simulink model "APSv3"  (R2020b)
settings: Solver=FixedStepDiscrete  StartTime=0.0  StopTime=Tmax  FixedStep=Ts  RelTol=1e-3
PreLoadFcn:
  | ROSconfig
  | wptsSignalSetup
PostLoadFcn:
  | configParameters
InitFcn:
  | configParameters
StartFcn:
  | gazeboSetup
StopFcn:
  | gazeboReset
  | goalreset
  | loadResults
model workspace (MAT data in the model file):
  idx = 1
  y = Simulink.Parameter
  y.DataType = 'auto'
  y.Dimensions = [0 0]
values from neighbouring files (symbols this model uses):
  distError = sqrt((initX^2)+(initY^2))    [config_APS_Turb.m]
  dynamicPlume = 0    [config_APS_Turb.m]
  init = [initX - 5,initY]    [config_APS_Turb.m]
  MaxC = max(max(max(PlumeD)))    [config_APS_Turb.m]
  N = 8    [config_APS_Turb.m]
  n = [n; i*(2*pi/N)]    [config_APS_Turb.m]
  Res = 1    [config_APS_Turb.m]
  Shrink = 1/Expand    [config_APS_Turb.m]
undefined symbols (not defined in the file or in its folder): angmax, Angular, concDetectionAccuracy, DiscIntNeverNeededParam, distThresh, Expand, get, hot, Kd, Ki, Kp, LimitSize, Linear, OffsetY, PlumeD, ResX, ResY, sensorDist, sourceAccuracy, T, Tmax, Ts, vmax, wgain
libraries: simulink x18, dspindex x8, dspswit3 x6, robotlib x3, dspsnks4 x3, sm_lib x2, nesl_utility x1, dspsigops x1, mobileRoboticsLib x1
(part 1 of 2)
PauseFcn:
  | gazeboPause
settings Model: OrderedModelArguments=off  Creator=ty  LastModifiedBy=Tyreeses'
settings SolverCC: AlgebraicLoopSolver=LineSearch
settings DataIOCC: ExternalInput=[r, b]  SaveFormat=Array  SaveState=on  InspectSignalLogs=on  ReturnWorkspaceOutputs=off  StateSaveName=wpts
settings DebuggingCC: ArithmeticOperatorsInVariantConditions=warning
settings SFSimCC: SimUseLocalCustomCode=off  CustomCodeUndefinedFunction=UseInterfaceOnly
settings RTWCC: RTWUseLocalCustomCode=off
settings SimMechanicsCC: VisOnUpdateDiagram=on  VisDuringSimulation=on  DefaultBodyColor=[.877 0 0]
settings ExplorerConfigSet: SimMechanicsOpenEditorOnUpdate=off  InternalSimMechanicsExplorerSettings="<ExplorerConfiguration><canonicalview>default</canonicalview><AnimationSetting><BasePlaybackSpeed>1.0</BasePlaybackSpeed><PlaybackSpeedFactor>4.0</PlaybackSpeedFactor></AnimationSetting><TilePanel><TileInfo><Tiles Columns=\"2\" Count=\"4\" Rows=\"2\"><Column Weight=\"0.5\"/><Column Weight=\"0.5\"/><Row Weight=\"0.5\"/><Row Weight=\"0.5\"/><Tile Height=\"1\" Width=\"1\" X=\"0\" Y=\"0\"/><Tile Height=\"1\" Width=\"1\" X=\"0\" Y=\"1\"/><Tile Height=\"1\" Width=\"1\" X=\"1\" Y=\"0\"/><Tile Height=\"1\" Width=\"1\" X=\"1\" Y=\"1\"/></Tiles></TileInfo><SceneInfo><SceneViewer><BGColor><R>0.60000002384185791</R><G>0.60000002384185791</G><B>0.60000002384185791</B></BGColor><Camera><DoPerspective>off</DoPerspective><Position><X>0.523539858098702515</X><Y>-0.526832295844210763</Y><Z>1.31558763938248235</Z></Position><Center><X>0.523539858098702515</X><Y>-0.526832295844210763</Y><Z>0.315587639382482354</Z></Center><Up><X>0</X><Y>1</Y><Z>-0</Z></Up><ViewLimDist>1</ViewLimDist><YLim>8.09056691591361421</YLim><XLim>11.4549610789668002</XLim></Camera></SceneViewer><SceneViewer><BGColor><R>0.60000002384185791</R><G>0.60000002384185791</G><B>0.60000002384185791</B></BGColor><Camera><DoPerspective>off</DoPerspective><Position><X>-1.00000000034924597</X><Y>-0.123102183445061519</Y><Z>0.275798201199813964</Z></Position><Center><X>-3.49245965480804443e-10</X><Y>-0.123102183445061519</Y><Z>0.275798201199813964</Z></Center><Up><X>0</X><Y>0</Y><Z>1</Z></Up><ViewLimDist>1</ViewLimDist><YLim>3.47753295219900371</YLim><XLim>4.92363576400452985</XLim></Camera></SceneViewer><SceneViewer><BGColor><R>0.60000002384185791</R><G>0.60000002384185791</G><B>0.60000002384185791</B></BGColor><Camera><DoPerspective>off</DoPerspective><Position><X>0.692144908773628886</X><Y>-0.692774488443842151</Y><Z>0.641997243049143074</Z></Position><Center><X>0.114794639584003433</X><Y>-0.115424219254216046</Y><Z>0.0646469738595174259</Z></Center><Up><X>-0.408248290463863073</X><Y>0.408248290463863073</Y><Z>0.816496580927726145</Z></Up><ViewLimDist>1</ViewLimDist><YLim>6.0070720394774666</YLim><XLim>8.50506239252750262</XLim></Camera></SceneViewer><SceneViewer><BGColor><R>0.60000002384185791</R><G>0.60000002384185791</G><B>0.60000002384185791</B></BGColor><Camera><DoPerspective>off</DoPerspective><Position><X>0.0489598554332313918</X><Y>-0.287272213681231237</Y><Z>1.31558770067272501</Z></Position><Center><X>0.0489598554332313918</X><Y>-0.287272213681231237</Y><Z>0.315587700672725013</Z></Center><Up><X>0</X><Y>1</Y><Z>-0</Z></Up><ViewLimDist>1</ViewLimDist><YLim>2.42704539801906094</YLim><XLim>3.4363118011556999</XLim></Camera></SceneViewer></SceneInfo></TilePanel><MechEditorPanel><Cameras><Camera><Id>Camera1</Id><Value><Name>TopCamera1</Name><NativeCamera><PositionKeyframeSet><Keyframe><Time>+0.0000000000000000e+00</Time><Value><X>+2.1442706964244174e-01</X><Y>+2.3082412087368320e-01</Y><Z>+8.5801428178680403e+00</Z></Value></Keyframe></PositionKeyframeSet><CenterKeyframeSet><Keyframe><Time>+0.0000000000000000e+00</Time><Value><X>+1.7666087274208450e-01</X><Y>+1.6219238056249624e-01</Y><Z>+3.9566976367888529e-01</Z></Value></Keyframe></CenterKeyframeSet><UpVectorKeyframeSet><Keyframe><Time>+0.0000000000000000e+00</Time><Value><X>-1.4536948631457236e-02</X><Y>+9.9985973958876295e-01</Y><Z>-8.3173477730344968e-03</Z></Value></Keyframe></UpVectorKeyframeSet></NativeCamera></Value></Camera></Cameras><GfxPanelCameraMap/><VideoCreator><PlaybackSpeedRatio>1.0</PlaybackSpeedRatio><FrameRate>30</FrameRate><VideoFormat>Motion JPEG AVI</VideoFormat><FrameSize>auto</FrameSize></VideoCreator></MechEditorPanel></ExplorerConfiguration>"

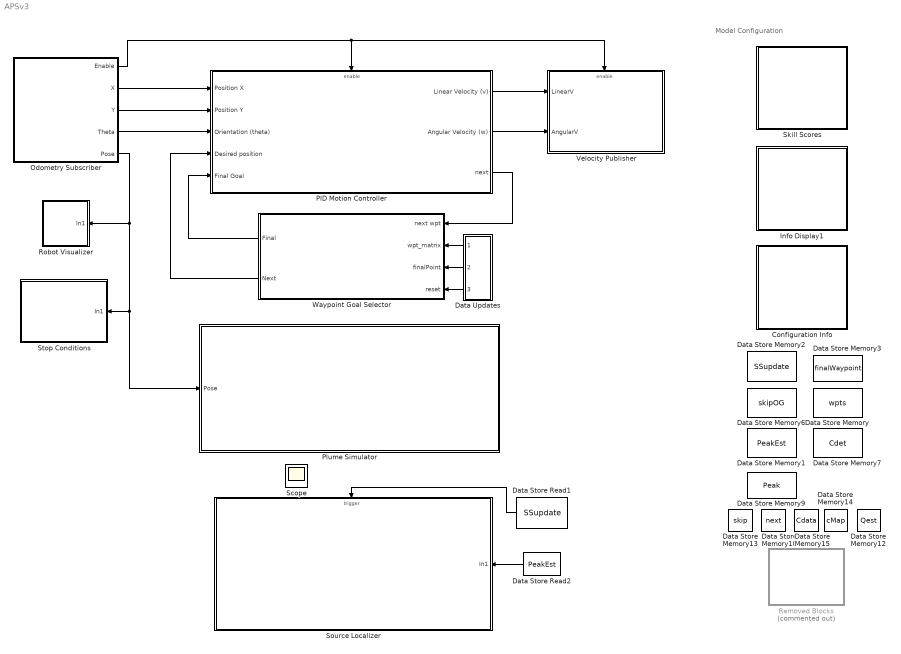
== system APSv3 ==
  note: Model Configuration
  Configuration Info : Subsystem
  Data Store Memory : DataStoreMemory  DataStoreName=wpts  ReadBeforeWriteMsg=warning  WriteAfterWriteMsg=warning  WriteAfterReadMsg=warning  InitialValue=waypoints  VectorParams1D=off  ShowAdditionalParam=off
  Data Store Memory1 : DataStoreMemory  DataStoreName=PeakEst  ReadBeforeWriteMsg=warning  WriteAfterWriteMsg=warning  WriteAfterReadMsg=warning  InitialValue=[25 25]  VectorParams1D=off  ShowAdditionalParam=off
  Data Store Memory10 : DataStoreMemory  DataStoreName=next  ReadBeforeWriteMsg=warning  WriteAfterWriteMsg=warning  WriteAfterReadMsg=warning  ShowAdditionalParam=off
  Data Store Memory12 : DataStoreMemory  DataStoreName=Qest  ReadBeforeWriteMsg=warning  WriteAfterWriteMsg=warning  WriteAfterReadMsg=warning  ShowAdditionalParam=off
  Data Store Memory13 : DataStoreMemory  DataStoreName=skip  ReadBeforeWriteMsg=warning  WriteAfterWriteMsg=warning  WriteAfterReadMsg=warning  ShowAdditionalParam=off
  Data Store Memory14 : DataStoreMemory  DataStoreName=cMap  ReadBeforeWriteMsg=warning  WriteAfterWriteMsg=warning  WriteAfterReadMsg=warning  InitialValue=zeros(size(PlumeD,1),size(PlumeD,2))  VectorParams1D=off  ShowAdditionalParam=off
  Data Store Memory15 : DataStoreMemory  DataStoreName=Cdata  ReadBeforeWriteMsg=warning  WriteAfterWriteMsg=warning  WriteAfterReadMsg=warning  InitialValue=ones(N+1,1)  ShowAdditionalParam=off  OutDataTypeStr=double
  Data Store Memory2 : DataStoreMemory  DataStoreName=SSupdate  ReadBeforeWriteMsg=warning  WriteAfterWriteMsg=warning  WriteAfterReadMsg=warning  InitialValue=1  ShowAdditionalParam=off  OutDataTypeStr=boolean
  Data Store Memory3 : DataStoreMemory  DataStoreName=finalWaypoint  ReadBeforeWriteMsg=warning  WriteAfterWriteMsg=warning  WriteAfterReadMsg=warning  InitialValue=finalPoint  ShowAdditionalParam=off  OutDataTypeStr=double
  Data Store Memory6 : DataStoreMemory  DataStoreName=skipOG  ReadBeforeWriteMsg=warning  WriteAfterWriteMsg=warning  WriteAfterReadMsg=warning  ShowAdditionalParam=off
  Data Store Memory7 : DataStoreMemory  DataStoreName=Cdet  ReadBeforeWriteMsg=warning  WriteAfterWriteMsg=warning  WriteAfterReadMsg=warning  ShowAdditionalParam=off
  Data Store Memory9 : DataStoreMemory  DataStoreName=Peak  ReadBeforeWriteMsg=warning  WriteAfterWriteMsg=warning  WriteAfterReadMsg=warning  InitialValue=[0,0]  ShowAdditionalParam=off
  Data Store Read1 : DataStoreRead  DataStoreName=SSupdate
  Data Store Read2 : DataStoreRead  DataStoreName=PeakEst
  Data Updates : Subsystem
  Info Display1 : Subsystem
  Odometry Subscriber : Subsystem
  PID Motion Controller : Subsystem
  Plume Simulator : Subsystem
  Removed Blocks : Subsystem  Commented=on
  Robot Visualizer : Subsystem
  Skill Scores : Subsystem
  Source Localizer : Subsystem  TreatAsAtomicUnit=on
  Stop Conditions : Subsystem
  Velocity Publisher : Subsystem
  Waypoint Goal Selector : Subsystem
  Scope : Scope
  wires:
  PID Motion Controller/1(Linear Velocity (v)) -> Velocity Publisher/1(LinearV)
  PID Motion Controller/2(Angular Velocity (w)) -> Velocity Publisher/2(AngularV)
  PID Motion Controller/3(next) -> Waypoint Goal Selector/1(next wpt)
  Waypoint Goal Selector/1(Final) -> PID Motion Controller/5(Final Goal)
  Waypoint Goal Selector/2(Next) -> PID Motion Controller/4(Desired position)
  Data Store Read2/1 -> Source Localizer/1(In1)
  Data Store Read1/1 -> Source Localizer/Trigger
  Data Updates/1(Out1) -> Waypoint Goal Selector/2(wpt_matrix)
  Data Updates/2(Out2) -> Waypoint Goal Selector/3(finalPoint)
  Data Updates/3(Out3) -> Waypoint Goal Selector/4(reset)
  Odometry Subscriber/1(Enable) -> Velocity Publisher/Enable, PID Motion Controller/Enable
  Odometry Subscriber/5(Pose) -> Plume Simulator/1(Pose), Stop Conditions/1(In1), Robot Visualizer/1(In1)
  Odometry Subscriber/2(X) -> PID Motion Controller/1(Position X)
  Odometry Subscriber/3(Y) -> PID Motion Controller/2(Position Y)
  Odometry Subscriber/4(Theta) -> PID Motion Controller/3(Orientation (theta))

== system APSv3/Configuration Info ==
  note: Nodes :
      | Publishers:
      | /sim_p3at/cmd_vel
      | /toggle_led
      | Subscribers:
      | /sim_p3at/odom
      | Messages:
      | geometry_msgs/Twist
      | std_msgs/Empty
  note: Startup Programs :
      | roscore
      | roslaunch nre_p3at p3at.gazebo.launch (starts Gazebo and /sim_p3at Nodes)
      | Arduino: ledtest3.ino
      | rosrun rosserial_python serial_node.py /dev/ttyACM0
      | MATLAB: (Simulink project)
  note: SS Parameters :
      | Expansion Constant: 2
  note: Plume Parameters :
      |
      | Diffusion constant (m2/s): c_diff = .8
      |
      | Advection velocity values (m/s): ux = 0 uy = 0 uz = 0.2
      |
      | Simulation Time (seconds): T = 10
      |
      | Domain dimensions (meters): L = 50 B = 50 H = 5
  "Counter " : Subsystem  Commented=on
  Floating Scope : Scope  Commented=on
      settings: Floating=on
  MechanismConfiguration : sm_lib/Utilities/Mechanism Configuration  UniformGravity=Constant  GravityVector=[0 0 -9.80665]  GravityUnits=m/s^2  LinearizationDelta=0.01
  Solver Configuration : nesl_utility/Solver Configuration  PhysicalDomain=network_engine_domain  SubClassName=solver  LeftPortType=input  RightPortType=generic  Accelerate=off  Tones=[]  Harmonics=[]  SimulateNoise=off  Profile=off  UseLocalSampling=off  EnableSwitchedLinearOptims=on  FrequencyDomain=off  UseCCode=off  RelTol=0.001  AbsTol=1e-06  MinStep=1e-09  ToWorkspace=off  RevertToSquareIcSolve=off  NumHomotopyIterations=100  PhasorMode=off  PhasorModeNumHarmonics=1  DoDC=on  ResidualTolerance=1e-09  UseLocalSolver=on  LocalSolverChoice=NE_BACKWARD_EULER_ADVANCER  LocalSolverSampleTime=Ts  DoFixedCost=on  MaxNonlinIter=3  MaxModeIter=2  LinearAlgebra=Sparse  DelaysMemoryBudget=1024  AutomaticFiltering=on  FilteringTimeConstant=0.01
  World : sm_lib/Frames and Transforms/World Frame
  connections:
  MechanismConfiguration/RConn1 -- World/RConn1 -- Solver Configuration/RConn1

== system APSv3/Data Updates ==
  Data Store Read : DataStoreRead  DataStoreName=wpts
  Data Store Read3 : DataStoreRead  DataStoreName=finalWaypoint
  Data Store Read5 : DataStoreRead  DataStoreName=SSupdate
  Data Store Write1 : DataStoreWrite  DataStoreName=finalWaypoint
  Demux : Demux  Outputs=2
  Probe : Probe  ProbeWidth=off  ProbeSampleTime=off  ProbeComplexSignal=off  ProbeSignalDimensions=on
  Terminator : Terminator
  Out1 : Outport  VectorParamsAs1DForOutWhenUnconnected=off
  Out2 : Outport  Port=2  VectorParamsAs1DForOutWhenUnconnected=off
  Out3 : Outport  Port=3  VectorParamsAs1DForOutWhenUnconnected=off
  wires:
  Data Store Read3/1 -> Out2/1
  Data Store Read/1 -> Out1/1, Probe/1
  Probe/1 -> Demux/1
  Demux/1 -> Data Store Write1/1
  Demux/2 -> Terminator/1
  Data Store Read5/1 -> Out3/1

== system APSv3/Info Display1 ==
  Clock : Clock
      settings: Decimation=2
  Constant : Constant  Value=[0 OffsetY]
  Constant1 : Constant  Value=MaxC
  Data Store Read : DataStoreRead  DataStoreName=PeakEst
  Data Store Read1 : DataStoreRead  DataStoreName=Peak
  Data Store Read3 : DataStoreRead  DataStoreName=Cdet
  Data Store Read4 : DataStoreRead  DataStoreName=Qest
  Detected Concentration Levels : DashboardScope  ShowInitialText=off  Ymin=0  Ymax=1000
  Display{,1..5} (6 alike) : Display
  Localization Error : DashboardScope  Ymin=0  Ymax=1.25  LegendPosition=Hide
  Sum1 : Sum
  To Workspace : ToWorkspace  VariableName=Tm  SampleTime=-1
      settings: MaxDataPoints=100
  wires:
  Data Store Read1/1 -> Display/1
  Data Store Read/1 -> Sum1/1
  Data Store Read4/1 -> Display3/1
  Constant1/1 -> Display2/1
  Clock/1 -> To Workspace/1, Display1/1
  Data Store Read3/1 -> Display5/1
  Constant/1 -> Sum1/2
  Sum1/1 -> Display4/1

== system APSv3/Odometry Subscriber ==
  Odometry Conversion : Subsystem
  Subscribe1 : robotlib/Subscribe  SourceLibraryInfo=This block requires Robotics System Toolbox  topicSource=Select from ROS network  topic=/sim_p3at/odom  messageType=nav_msgs/Odometry  sampleTime=-1  messageQueueLength=51
  Enable : Outport  VectorParamsAs1DForOutWhenUnconnected=off
  X : Outport  Port=2  VectorParamsAs1DForOutWhenUnconnected=off
  Y : Outport  Port=3  VectorParamsAs1DForOutWhenUnconnected=off
  Theta : Outport  Port=4  VectorParamsAs1DForOutWhenUnconnected=off
  Pose : Outport  Port=5  VectorParamsAs1DForOutWhenUnconnected=off
  wires:
  Subscribe1/1 -> Enable/1
  Subscribe1/2 -> Odometry Conversion/1(In1)
  Odometry Conversion/3(Out3) -> Theta/1
  Odometry Conversion/4(pose) -> Pose/1
  Odometry Conversion/1(<X>) -> X/1
  Odometry Conversion/2(<Y>) -> Y/1

== system APSv3/PID Motion Controller ==
  Position X : Inport
  Position Y : Inport  Port=2
  Orientation (theta) : Inport  Port=3
  Desired position : Inport  Port=4
  Final Goal : Inport  Port=5
  Enable : EnablePort
  Compare To Zero1 : simulink/Logic and Bit Operations/Compare To Zero  relop=>  OutDataTypeStr=boolean
  Constant3 : Constant  Value=0
  Data Store Write : DataStoreWrite  DataStoreName=SSupdate
  Data Store Write1 : DataStoreWrite  DataStoreName=next
  Initialize Goal : Subsystem
  PID Calculations : Subsystem
  Switch1 : Switch  Criteria=u2 ~= 0
  Linear Velocity (v) : Outport  VectorParamsAs1DForOutWhenUnconnected=off
  Angular Velocity (w) : Outport  Port=2  VectorParamsAs1DForOutWhenUnconnected=off
  next : Outport  Port=3  VectorParamsAs1DForOutWhenUnconnected=off
  wires:
  Switch1/1 -> Angular Velocity (w)/1
  Compare To Zero1/1 -> Data Store Write1/1, next/1
  Constant3/1 -> Switch1/1
  Final Goal/1 -> Data Store Write/1
  PID Calculations/2(Out2) -> Compare To Zero1/1, Switch1/2
  Desired position/1 -> Initialize Goal/1(In1)  "SP"
  Position Y/1 -> PID Calculations/2(In2)
  Position X/1 -> PID Calculations/3(In3)
  Orientation (theta)/1 -> PID Calculations/4(In4)
  PID Calculations/1(Out1) -> Linear Velocity (v)/1
  PID Calculations/3(Out3) -> Switch1/3
  Initialize Goal/1(Out1) -> PID Calculations/1(SP)

== system APSv3/Plume Simulator ==
  Pose : Inport
  C(t,x,y) : Subsystem
  Peak Selector : Subsystem
  Plume Model Data Simulator : Subsystem
  Terminator : Terminator
  Terminator1 : Terminator
  wires:
  C(t,x,y)/1(z(t)) -> Peak Selector/1(In1)
  Peak Selector/2(Peak C) -> Terminator1/1
  Peak Selector/1(Peak Pose) -> Terminator/1
  Pose/1 -> Plume Model Data Simulator/1(In2)
  Plume Model Data Simulator/2(t) -> C(t,x,y)/2(time)
  Plume Model Data Simulator/1(C) -> C(t,x,y)/1(c)
  Plume Model Data Simulator/3(MaxPose) -> C(t,x,y)/3(In1)

== system APSv3/Removed Blocks ==
  Constant3 : Constant  Value=MaxC
  Data Store Memory11 : DataStoreMemory  DataStoreName=locError  ReadBeforeWriteMsg=warning  WriteAfterWriteMsg=warning  WriteAfterReadMsg=warning  ShowAdditionalParam=off
  Data Store Memory16 : DataStoreMemory  DataStoreName=finalPoint  ReadBeforeWriteMsg=warning  WriteAfterWriteMsg=warning  WriteAfterReadMsg=warning  ShowAdditionalParam=off
  Data Store Memory4 : DataStoreMemory  DataStoreName=OG  ReadBeforeWriteMsg=warning  WriteAfterWriteMsg=warning  WriteAfterReadMsg=warning  InitialValue=[0 0]  ShowAdditionalParam=off
  Data Store Memory5 : DataStoreMemory  DataStoreName=DT  ReadBeforeWriteMsg=warning  WriteAfterWriteMsg=warning  WriteAfterReadMsg=warning  InitialValue=[0]  VectorParams1D=off  ShowAdditionalParam=off
  Data Store Memory8 : DataStoreMemory  DataStoreName=Cmax  ReadBeforeWriteMsg=warning  WriteAfterWriteMsg=warning  WriteAfterReadMsg=warning  InitialValue=MaxC  ShowAdditionalParam=off
  Display2 : Display  Commented=on
  Dynamic Plume Concentrations : Subsystem  Commented=on
  Gain : Gain  Commented=on  Gain=1/Ts
  Rounding Function2 : Rounding  Commented=on  Operator=ceil
  Saturation : Saturate  Commented=on  UpperLimit=T/Ts  LowerLimit=1
  Subsystem : Subsystem  Commented=on
  Terminator : Terminator  Commented=on
  To Workspace3 : ToWorkspace  VariableName=Cmax1  SaveFormat=Timeseries  SampleTime=-1
  wires:
  Gain/1 -> Rounding Function2/1
  Dynamic Plume Concentrations/1(peak) -> Subsystem/1(In1)
  Saturation/1 -> Dynamic Plume Concentrations/1(DT)
  Dynamic Plume Concentrations/2(plume) -> Terminator/1
  Subsystem/1(Out1) -> Display2/1
  Rounding Function2/1 -> Saturation/1  "u"
  Constant3/1 -> To Workspace3/1

== system APSv3/Robot Visualizer ==
  In1 : Inport
  Constant1 : Constant
  Current Origin : dspindex/Variable Selector  NumInputs=1  rowsOrCols=Rows  IdxMode=Variable  Elements=[1 3]  ZerOneIdxMode=One-based  errmode=Clip Index  FillMode=off  FillValues=0
  Data Store Read : DataStoreRead  DataStoreName=next
  Data Store Read4 : DataStoreRead  DataStoreName=wpts
  Robot Visualizer : mobileRoboticsLib/Environments/Robot Visualizer  Priority=99  robotRadius=.34  mapName=gasMap  showTrajectory=on  hasWaypoints=on  hasLidar=off  sensorOffset=[ 0 0 ]  scanAngles=0  hasObjDetector=off  objDetectorOffset=[ 0,0 ]  objDetectorAngle=0  objDetectorFOV=0  objDetectorMaxRange=0  objectColors=[1,0,0;0,1,0;0,0,1]  objectMarkers='s'
  To Workspace : ToWorkspace  VariableName=goalpoints  SampleTime=-1
      settings: Save2DSignal=2-D array (concatenate along first dimension)
  Triggered To Workspace : dspsnks4/Triggered To Workspace  TriggerType=Rising edge  VariableName=pathUpdates  Buffer=1000  Save2DMode=3-D array (concatenate along third dimension)
      settings: SourceProductBaseCode=DS  FixptAsFi=off
  wires:
  In1/1 -> Robot Visualizer/1
  Data Store Read4/1 -> To Workspace/1, Current Origin/1, Robot Visualizer/2
  Data Store Read/1 -> Triggered To Workspace/Trigger
  Constant1/1 -> Current Origin/2
  Current Origin/1 -> Triggered To Workspace/1

== system APSv3/Skill Scores ==
  Location Estimate (SL) : Subsystem
  Source Estimate (SQ) : Subsystem

== system APSv3/Source Localizer ==
  In1 : Inport
  Trigger : TriggerPort  VariantControl=Variant  InitialTriggerSignalState=positive  PortDimensions=1
  Data Store Read : DataStoreRead  DataStoreName=wpts
  Data Store Write : DataStoreWrite  DataStoreName=wpts
  Path Search Update : Subsystem
  wires:
  Data Store Read/1 -> Path Search Update/1(In1)
  In1/1 -> Path Search Update/2(In2)
  Path Search Update/1(Out1) -> Data Store Write/1

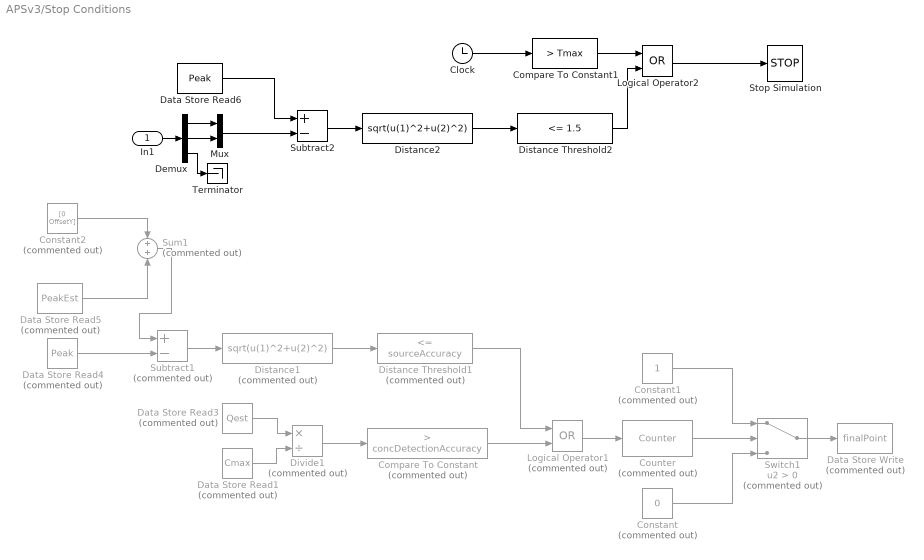
== system APSv3/Stop Conditions ==
  In1 : Inport
  Clock : Clock
  Compare To Constant : simulink/Logic and Bit Operations/Compare To Constant  Commented=on  relop=>  const=concDetectionAccuracy  OutDataTypeStr=boolean
  Compare To Constant1 : simulink/Logic and Bit Operations/Compare To Constant  relop=>  const=Tmax  OutDataTypeStr=boolean
  Constant : Constant  Commented=on  Value=0
  Constant1 : Constant  Commented=on
  Constant2 : Constant  Commented=on  Value=[0 OffsetY]
  Counter : dspswit3/Counter  Commented=on  Direction=Up  CountEvent=Rising edge  CounterSize=User defined  MaxCount=255  InitialCount=0  Output=Count  HitValue=32  ResetInput=off  SamplesPerFrame=1  Ts=1  CntDtype=double  HitDtype=Logical
  Data Store Read1 : DataStoreRead  Commented=on  DataStoreName=Cmax
  Data Store Read3 : DataStoreRead  Commented=on  DataStoreName=Qest
  Data Store Read4 : DataStoreRead  Commented=on  DataStoreName=Peak
  Data Store Read5 : DataStoreRead  Commented=on  DataStoreName=PeakEst
  Data Store Read6 : DataStoreRead  DataStoreName=Peak
  Data Store Write : DataStoreWrite  Commented=on  DataStoreName=finalPoint
  Demux : Demux  Outputs=3
  Distance Threshold1 : simulink/Logic and Bit Operations/Compare To Constant  Commented=on  relop=<=  const=sourceAccuracy  OutDataTypeStr=boolean
  Distance Threshold2 : simulink/Logic and Bit Operations/Compare To Constant  relop=<=  const=1.5  OutDataTypeStr=boolean
  Distance1 : Fcn  Commented=on  Expr=sqrt(u(1)^2+u(2)^2)
  Distance2 : Fcn  Expr=sqrt(u(1)^2+u(2)^2)
  Divide1 : Product  Commented=on  Inputs=*/
  Logical Operator1 : Logic  Commented=on  Operator=OR  AllPortsSameDT=off  OutDataTypeStr=boolean
  Logical Operator2 : Logic  Operator=OR  AllPortsSameDT=off  OutDataTypeStr=boolean
  Mux : Mux  Inputs=2
  Stop Simulation : Stop
  Subtract1 : Sum  Commented=on  Inputs=+-
  Subtract2 : Sum  Inputs=+-
  Sum1 : Sum  Commented=on
  Switch1 : Switch  Commented=on  Criteria=u2 > Threshold
  Terminator : Terminator
  wires:
  Logical Operator1/1 -> Counter/1
  Compare To Constant/1 -> Logical Operator1/2
  Data Store Read3/1 -> Divide1/1
  Data Store Read5/1 -> Sum1/2
  Subtract1/1 -> Distance1/1
  Distance Threshold1/1 -> Logical Operator1/1
  Data Store Read4/1 -> Subtract1/2
  Data Store Read1/1 -> Divide1/2
  Distance1/1 -> Distance Threshold1/1
  Divide1/1 -> Compare To Constant/1
  Data Store Read6/1 -> Subtract2/1
  Subtract2/1 -> Distance2/1
  Distance2/1 -> Distance Threshold2/1
  Distance Threshold2/1 -> Logical Operator2/2
  Constant1/1 -> Switch1/1
  Constant/1 -> Switch1/3
  Counter/1 -> Switch1/2
  Switch1/1 -> Data Store Write/1
  In1/1 -> Demux/1
  Demux/1 -> Mux/1
  Demux/2 -> Mux/2
  Mux/1 -> Subtract2/2
  Demux/3 -> Terminator/1
  Constant2/1 -> Sum1/1
  Sum1/1 -> Subtract1/1
  Compare To Constant1/1 -> Logical Operator2/1
  Clock/1 -> Compare To Constant1/1
  Logical Operator2/1 -> Stop Simulation/1

== system APSv3/Velocity Publisher ==
  LinearV : Inport
  AngularV : Inport  Port=2
  Enable : EnablePort
  Blank Message : robotlib/Blank Message  SourceLibraryInfo=This block requires Robotics System Toolbox  messageType=geometry_msgs/Twist  SampleTime=-1
  Bus Assignment : BusAssignment  DialogController=Simulink.DDGSource_BusAssignment  AssignedSignals=Linear.X,Angular.Z
  Publish1 : robotlib/Publish  SourceLibraryInfo=This block requires Robotics System Toolbox  topicSource=Select from ROS network  topic=/sim_p3at/cmd_vel  messageType=geometry_msgs/Twist  messageQueueLength=105
  wires:
  AngularV/1 -> Bus Assignment/3
  Bus Assignment/1 -> Publish1/1
  LinearV/1 -> Bus Assignment/2
  Blank Message/1 -> Bus Assignment/1

== system APSv3/Waypoint Goal Selector ==
  next wpt : Inport
  wpt_matrix : Inport  Port=2
  finalPoint : Inport  Port=3
  reset : Inport  Port=4
  "Counter " : Subsystem
  Current Goal Selector : dspindex/Variable Selector  NumInputs=1  rowsOrCols=Rows  IdxMode=Variable  Elements=[1 3]  ZerOneIdxMode=One-based  errmode=Clip Index  FillMode=off  FillValues=0
  Data Store Read : DataStoreRead  DataStoreName=skipOG
  Relational Operator : RelationalOperator  Operator===  OutDataTypeStr=boolean  RndMeth=Simplest
  Skip Conditions : Subsystem
  Sum : Sum  Inputs=|++
  Final : Outport  VectorParamsAs1DForOutWhenUnconnected=off
  Next : Outport  Port=2  VectorParamsAs1DForOutWhenUnconnected=off
  wires:
  wpt_matrix/1 -> Current Goal Selector/1
  Current Goal Selector/1 -> Next/1
  "Counter "/1(Out1) -> Sum/1
  next wpt/1 -> Skip Conditions/1(In1), "Counter "/1(In1)
  Relational Operator/1 -> Final/1
  finalPoint/1 -> Relational Operator/1
  reset/1 -> "Counter "/2(In2)
  Data Store Read/1 -> Sum/2
  Sum/1 -> Relational Operator/2, Current Goal Selector/2

== system APSv3/Configuration Info/Counter  ==
  In1 : Inport
  Counter : dspswit3/Counter  Direction=Up  CountEvent=Non-zero sample  CounterSize=User defined  MaxCount=255  InitialCount=0  Output=Count  HitValue=32  ResetInput=off  SamplesPerFrame=1  Ts=1  CntDtype=single  HitDtype=Logical
  Counter1 : dspswit3/Counter  Direction=Up  CountEvent=Rising edge  CounterSize=User defined  MaxCount=255  InitialCount=0  Output=Count  HitValue=32  ResetInput=off  SamplesPerFrame=1  Ts=1  CntDtype=double  HitDtype=Logical
  Detect Increase : simulink/Logic and Bit Operations/Detect Increase  vinit=0.0  OutDataTypeStr=boolean
  Out1 : Outport  VectorParamsAs1DForOutWhenUnconnected=off
  wires:
  In1/1 -> Counter/1
  Counter/1 -> Detect Increase/1
  Detect Increase/1 -> Counter1/1
  Counter1/1 -> Out1/1

== system APSv3/Odometry Subscriber/Odometry Conversion ==
  In1 : Inport
  Bus Selector3 : BusSelector  OutputSignals=Pose.Pose.Position.X,Pose.Pose.Position.Y,Pose.Pose.Orientation.X,Pose.Pose.Orientation.Y,Pose.Pose.Orientation.Z,Pose.Pose.Orientation.W
  Conversion : MATLAB Function  TreatAsAtomicUnit=on
  Mux : Mux  Inputs=3
  <X> : Outport  VectorParamsAs1DForOutWhenUnconnected=off
  <Y> : Outport  Port=2  VectorParamsAs1DForOutWhenUnconnected=off
  Out3 : Outport  Port=3  VectorParamsAs1DForOutWhenUnconnected=off
  pose : Outport  Port=4  VectorParamsAs1DForOutWhenUnconnected=off
  wires:
  In1/1 -> Bus Selector3/1
  Bus Selector3/3 -> Conversion/1(x)  "<X>"
  Bus Selector3/4 -> Conversion/2(y)  "<Y>"
  Bus Selector3/5 -> Conversion/3(z)  "<Z>"
  Bus Selector3/6 -> Conversion/4(w)  "<W>"
  Conversion/1(yaw) -> Mux/3, Out3/1
  Bus Selector3/2 -> Mux/2, <Y>/1  "<Y>"
  Bus Selector3/1 -> Mux/1, <X>/1  "<X>"
  Mux/1 -> pose/1  "pose"

== system APSv3/PID Motion Controller/Initialize Goal ==
  In1 : Inport
  Constant : Constant  Value=init
  Data Store Read : DataStoreRead  DataStoreName=skip
  Switch : Switch  Criteria=u2 > Threshold
  Out1 : Outport  VectorParamsAs1DForOutWhenUnconnected=off
  wires:
  Data Store Read/1 -> Switch/2
  In1/1 -> Switch/1
  Constant/1 -> Switch/3
  Switch/1 -> Out1/1

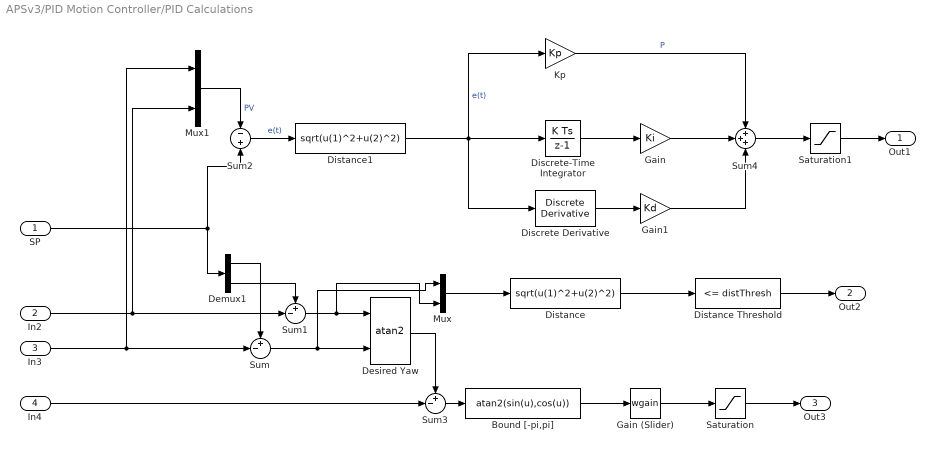
== system APSv3/PID Motion Controller/PID Calculations ==
  SP : Inport
  In2 : Inport  Port=2
  In3 : Inport  Port=3
  In4 : Inport  Port=4
  Bound [-pi,pi] : Fcn  Expr=atan2(sin(u),cos(u))
  Demux1 : Demux  Outputs=2
  Desired Yaw : Trigonometry  Operator=atan2
  Discrete Derivative : simulink/Discrete/Discrete Derivative  gainval=1  ICPrevScaledInput=0.0  OutMin=[]  OutMax=[]  OutDataType=fixdt(1, 16)  OutScaling=2^-10  DoSatur=off
  Discrete-Time Integrator : DiscreteIntegrator  gainval=1  SampleTime=-1  ICPrevOutput=DiscIntNeverNeededParam  ICPrevScaledInput=DiscIntNeverNeededParam
  Distance : Fcn  Expr=sqrt(u(1)^2+u(2)^2)
  Distance Threshold : simulink/Logic and Bit Operations/Compare To Constant  relop=<=  const=distThresh  OutDataTypeStr=boolean
  Distance1 : Fcn  Expr=sqrt(u(1)^2+u(2)^2)
  Gain : Gain  Gain=Ki
  Gain (Slider) : simulink/Math Operations/Slider Gain  gain=wgain  low=1  high=10
  Gain1 : Gain  Gain=Kd
  Kp : Gain  Gain=Kp
  Mux : Mux  Inputs=2
  Mux1 : Mux  Inputs=2
  Saturation : Saturate  UpperLimit=angmax  LowerLimit=-angmax
  Saturation1 : Saturate  UpperLimit=vmax  LowerLimit=-.5
  Sum : Sum  Inputs=+-|
  Sum1 : Sum  Inputs=+-|
  Sum2 : Sum  Inputs=-+
  Sum3 : Sum  Inputs=+-|
  Sum4 : Sum  Inputs=+++
  Out1 : Outport  VectorParamsAs1DForOutWhenUnconnected=off
  Out2 : Outport  Port=2  VectorParamsAs1DForOutWhenUnconnected=off
  Out3 : Outport  Port=3  VectorParamsAs1DForOutWhenUnconnected=off
  wires:
  In4/1 -> Sum3/2
  Desired Yaw/1 -> Sum3/1
  Sum/1 -> Desired Yaw/2, Mux/1
  Gain (Slider)/1 -> Saturation/1
  Saturation/1 -> Out3/1
  Sum3/1 -> Bound [-pi,pi]/1
  Mux1/1 -> Sum2/1  "PV"
  Kp/1 -> Sum4/1  "P"
  Distance1/1 -> Kp/1, Discrete-Time Integrator/1, Discrete Derivative/1  "e(t)"
  Discrete-Time Integrator/1 -> Gain/1
  Demux1/1 -> Sum/1
  Demux1/2 -> Sum1/1
  Sum1/1 -> Desired Yaw/1, Mux/2
  SP/1 -> Demux1/1, Sum2/2
  In2/1 -> Sum1/2, Mux1/2
  In3/1 -> Sum/2, Mux1/1
  Distance/1 -> Distance Threshold/1
  Mux/1 -> Distance/1
  Bound [-pi,pi]/1 -> Gain (Slider)/1
  Sum2/1 -> Distance1/1  "e(t)"
  Gain/1 -> Sum4/2
  Sum4/1 -> Saturation1/1
  Discrete Derivative/1 -> Gain1/1
  Gain1/1 -> Sum4/3
  Distance Threshold/1 -> Out2/1
  Saturation1/1 -> Out1/1

== system APSv3/Plume Simulator/C(t,x,y) ==
  c : Inport
  time : Inport  Port=2
  In1 : Inport  Port=3
  Bus Creator : BusCreator  Inputs=4
  Demux : Demux  Outputs=2
  Mux : Mux  Commented=on
      settings: DisplayOption=signals
  To File : ToFile  Commented=on  Filename=ConcentrationData.mat  MatrixName=ConcentrationMap  SaveFormat=Timeseries
  z(t) : Outport  VectorParamsAs1DForOutWhenUnconnected=off
  wires:
  Demux/1 -> Mux/1, Bus Creator/1
  Demux/2 -> Mux/2, Bus Creator/2
  Mux/1 -> To File/1
  time/1 -> Bus Creator/4, Mux/4
  Bus Creator/1 -> z(t)/1
  c/1 -> Bus Creator/3, Mux/3
  In1/1 -> Demux/1

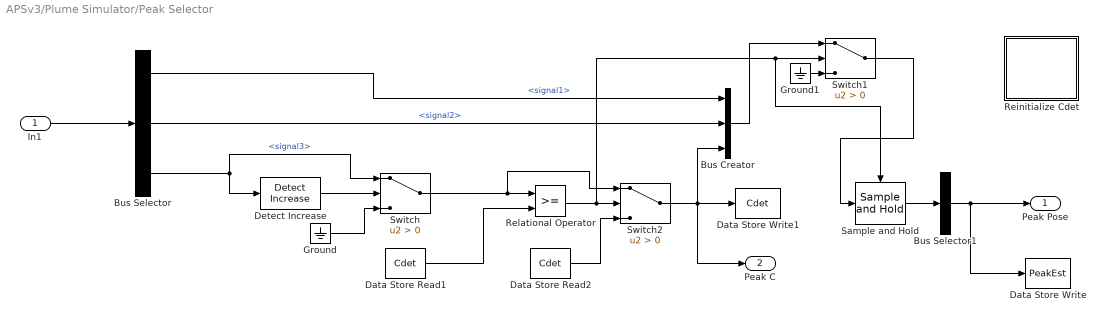
== system APSv3/Plume Simulator/Peak Selector ==
  In1 : Inport
  Bus Creator : BusCreator  Inputs=3
  Bus Selector : BusSelector  OutputSignals=signal1,signal2,signal3
  Bus Selector1 : BusSelector  OutputSignals=signal1,signal2  OutputAsBus=on
  Data Store Read1 : DataStoreRead  DataStoreName=Cdet
  Data Store Read2 : DataStoreRead  DataStoreName=Cdet
  Data Store Write : DataStoreWrite  DataStoreName=PeakEst
  Data Store Write1 : DataStoreWrite  DataStoreName=Cdet
  Detect Increase : simulink/Logic and Bit Operations/Detect Increase  vinit=0.0  OutDataTypeStr=boolean
  Ground : Ground
  Ground1 : Ground
  Reinitialize Cdet : Subsystem
  Relational Operator : RelationalOperator  OutDataTypeStr=boolean  RndMeth=Simplest
  Sample and Hold : dspsigops/Sample and Hold  trig=Rising edge  initCond=0  latchinput=off
  Switch : Switch  Criteria=u2 > Threshold
  Switch1 : Switch  Criteria=u2 > Threshold  OutDataTypeStr=double
  Switch2 : Switch  Criteria=u2 > Threshold
  Peak Pose : Outport  VectorParamsAs1DForOutWhenUnconnected=off
  Peak C : Outport  Port=2  VectorParamsAs1DForOutWhenUnconnected=off
  wires:
  Bus Selector/3 -> Detect Increase/1, Switch/1  "<signal3>"
  Detect Increase/1 -> Switch/2
  Ground/1 -> Switch/3
  Bus Selector/1 -> Bus Creator/1  "<signal1>"
  Bus Selector/2 -> Bus Creator/2  "<signal2>"
  In1/1 -> Bus Selector/1
  Switch/1 -> Switch2/1, Relational Operator/1
  Relational Operator/1 -> Switch1/2, Sample and Hold/Trigger, Switch2/2
  Data Store Read2/1 -> Switch2/3
  Switch2/1 -> Peak C/1, Data Store Write1/1, Bus Creator/3
  Switch1/1 -> Sample and Hold/1
  Bus Creator/1 -> Switch1/1
  Bus Selector1/1 -> Data Store Write/1, Peak Pose/1
  Ground1/1 -> Switch1/3
  Sample and Hold/1 -> Bus Selector1/1
  Data Store Read1/1 -> Relational Operator/2

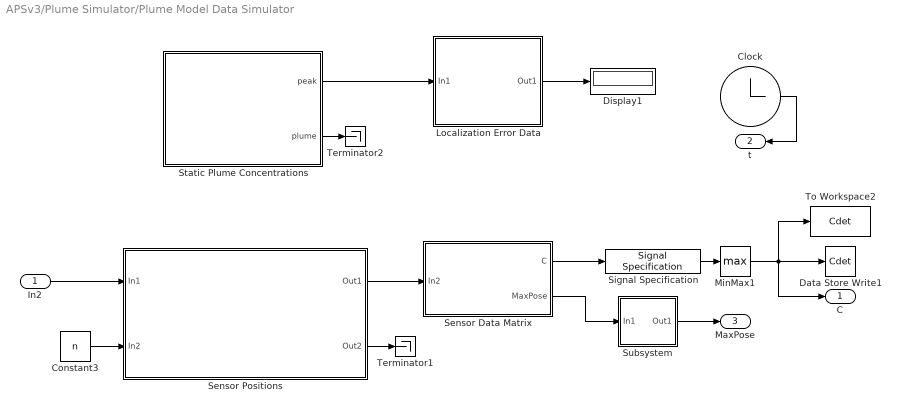
== system APSv3/Plume Simulator/Plume Model Data Simulator ==
  In2 : Inport
  Clock : Clock
      settings: Decimation=3
  Constant3 : Constant  Value=n
  Data Store Write1 : DataStoreWrite  DataStoreName=Cdet
  Display1 : Display
  Localization Error Data : Subsystem
  MinMax1 : MinMax  Function=max
  Sensor Data Matrix : Subsystem
  Sensor Positions : Subsystem
  Signal Specification : SignalSpecification  OutDataTypeStr=double  SampleTime=.01
  Static Plume Concentrations : Subsystem
  Subsystem : Subsystem
  Terminator1 : Terminator
  Terminator2 : Terminator
  To Workspace2 : ToWorkspace  VariableName=Cdet  SaveFormat=Timeseries  SampleTime=-1
  C : Outport  VectorParamsAs1DForOutWhenUnconnected=off
  t : Outport  Port=2  VectorParamsAs1DForOutWhenUnconnected=off
  MaxPose : Outport  Port=3  VectorParamsAs1DForOutWhenUnconnected=off
  wires:
  Clock/1 -> t/1
  Sensor Positions/1(Out1) -> Sensor Data Matrix/1(In2)
  MinMax1/1 -> C/1, To Workspace2/1, Data Store Write1/1
  Sensor Positions/2(Out2) -> Terminator1/1
  Sensor Data Matrix/1(C) -> Signal Specification/1
  Signal Specification/1 -> MinMax1/1
  In2/1 -> Sensor Positions/1(In1)
  Constant3/1 -> Sensor Positions/2(In2)
  Static Plume Concentrations/1(peak) -> Localization Error Data/1(In1)
  Static Plume Concentrations/2(plume) -> Terminator2/1
  Localization Error Data/1(Out1) -> Display1/1
  Sensor Data Matrix/2(MaxPose) -> Subsystem/1(In1)
  Subsystem/1(Out1) -> MaxPose/1

== system APSv3/Removed Blocks/Dynamic Plume Concentrations ==
  DT : Inport
  Constant : Constant  Value=OffsetY
  Constant1 : Constant  Value=T/Ts
  Constant2 : Constant  Value=dynamicPlume
  Data Store Write1 : DataStoreWrite  DataStoreName=Cmax
  Dynamic Plume Concentration Data : Constant  Value=PlumeD  VectorParams1D=off  OutDataTypeStr=double  LockScale=on
  Gain : Gain  Gain=1/100
  MATLAB Function : MATLAB Function  TreatAsAtomicUnit=on
  Matrix Viewer : dspsnks4/Matrix Viewer  Commented=on  ImageParams=off  CMapStr=hot(256)  AxisColorbar=on  AxisParams=off  AxisOrigin=Lower left corner  AxisTickMode=Auto  XTickRange=[0 1]  YTickRange=[0 1]  XLabel=X (quarter meters)  YLabel=Y (quarter meters)  ZLabel=Concentration  FigPos=[0 1750 500 400]  AxisZoom=off
      settings: SourceProductBaseCode=DS  YMin=0  YMax=1000
  Permute Dimensions1 : PermuteDimensions
  Switch : Switch  Criteria=u2 > Threshold
  To Workspace3 : ToWorkspace  VariableName=Cmax  SaveFormat=Timeseries  SampleTime=-1
  peak : Outport  VectorParamsAs1DForOutWhenUnconnected=off
  plume : Outport  Port=2  VectorParamsAs1DForOutWhenUnconnected=off
  wires:
  Dynamic Plume Concentration Data/1 -> MATLAB Function/1(PlumeD)
  MATLAB Function/2(Cmax) -> To Workspace3/1, Data Store Write1/1
  MATLAB Function/1(Plume) -> Gain/1, Permute Dimensions1/1
  Permute Dimensions1/1 -> plume/1
  MATLAB Function/3(Peak) -> peak/1
  DT/1 -> Switch/1
  Constant1/1 -> Switch/3
  Constant2/1 -> Switch/2
  Switch/1 -> MATLAB Function/2(u)
  Gain/1 -> Matrix Viewer/1
  Constant/1 -> MATLAB Function/3(OffsetY)

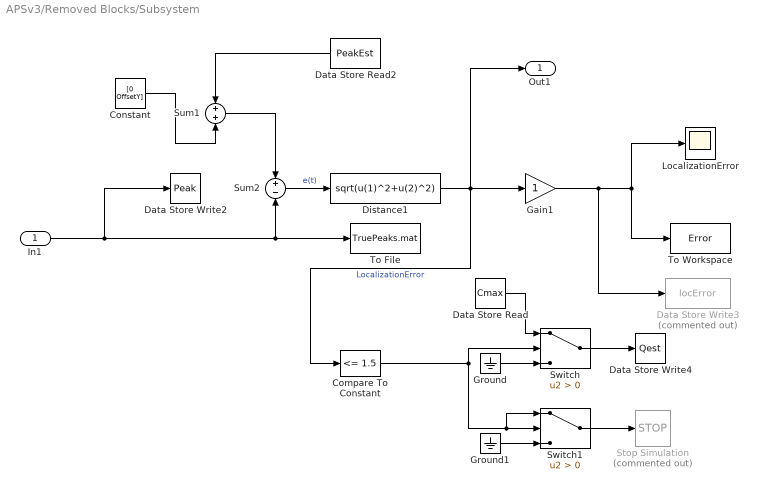
== system APSv3/Removed Blocks/Subsystem ==
  In1 : Inport
  Compare To Constant : simulink/Logic and Bit Operations/Compare To Constant  relop=<=  const=1.5  OutDataTypeStr=boolean
  Constant : Constant  Value=[0 OffsetY]
  Data Store Read : DataStoreRead  DataStoreName=Cmax
  Data Store Read2 : DataStoreRead  DataStoreName=PeakEst
  Data Store Write2 : DataStoreWrite  DataStoreName=Peak
  Data Store Write3 : DataStoreWrite  Commented=on  DataStoreName=locError
  Data Store Write4 : DataStoreWrite  DataStoreName=Qest
  Distance1 : Fcn  Expr=sqrt(u(1)^2+u(2)^2)
  Gain1 : Gain
  Ground : Ground
  Ground1 : Ground
  LocalizationError : Scope
  Stop Simulation : Stop  Commented=on
  Sum1 : Sum
  Sum2 : Sum  Inputs=+-
  Switch : Switch  Criteria=u2 > Threshold
  Switch1 : Switch  Criteria=u2 > Threshold
  To File : ToFile  Filename=TruePeaks.mat  MatrixName=ActualPeaks
      settings: Decimation=2
  To Workspace : ToWorkspace  VariableName=Error  SaveFormat=Timeseries  SampleTime=-1
  Out1 : Outport  VectorParamsAs1DForOutWhenUnconnected=off
  wires:
  Sum2/1 -> Distance1/1  "e(t)"
  Data Store Read2/1 -> Sum1/1
  Distance1/1 -> Out1/1, Compare To Constant/1, Gain1/1  "LocalizationError"
  In1/1 -> Data Store Write2/1, To File/1, Sum2/2
  Constant/1 -> Sum1/2
  Sum1/1 -> Sum2/1
  Gain1/1 -> Data Store Write3/1, To Workspace/1, LocalizationError/1
  Compare To Constant/1 -> Switch1/1, Switch1/2, Switch/2
  Ground/1 -> Switch/3
  Data Store Read/1 -> Switch/1
  Ground1/1 -> Switch1/3
  Switch1/1 -> Stop Simulation/1
  Switch/1 -> Data Store Write4/1

== system APSv3/Skill Scores/Location Estimate (SL) ==
  Data Store Read : DataStoreRead  DataStoreName=Peak
  Data Store Read2 : DataStoreRead  DataStoreName=PeakEst
  Distance : Fcn  Expr=sqrt(u(1)^2+u(2)^2)
  Gain : Gain  Gain=1/distError
  Subtract : Sum  Inputs=+-
  To Workspace1 : ToWorkspace  VariableName=ScoreL  SampleTime=-1
      settings: MaxDataPoints=100  Save2DSignal=2-D array (concatenate along first dimension)
  wires:
  Data Store Read/1 -> Subtract/2
  Subtract/1 -> Distance/1
  Data Store Read2/1 -> Subtract/1
  Distance/1 -> Gain/1
  Gain/1 -> To Workspace1/1

== system APSv3/Skill Scores/Source Estimate (SQ) ==
  Abs : Abs
  Constant : Constant  Value=MaxC
  Data Store Read : DataStoreRead  DataStoreName=Qest
  Divide : Product  Inputs=*/
  Q estimate : Subsystem
  Subtract1 : Sum  Inputs=-+
  To Workspace : ToWorkspace  VariableName=ScoreQ  SampleTime=-1
      settings: MaxDataPoints=100
  wires:
  Divide/1 -> Abs/1
  Subtract1/1 -> Divide/1
  Abs/1 -> To Workspace/1
  Data Store Read/1 -> Subtract1/1
  Constant/1 -> Divide/2, Subtract1/2

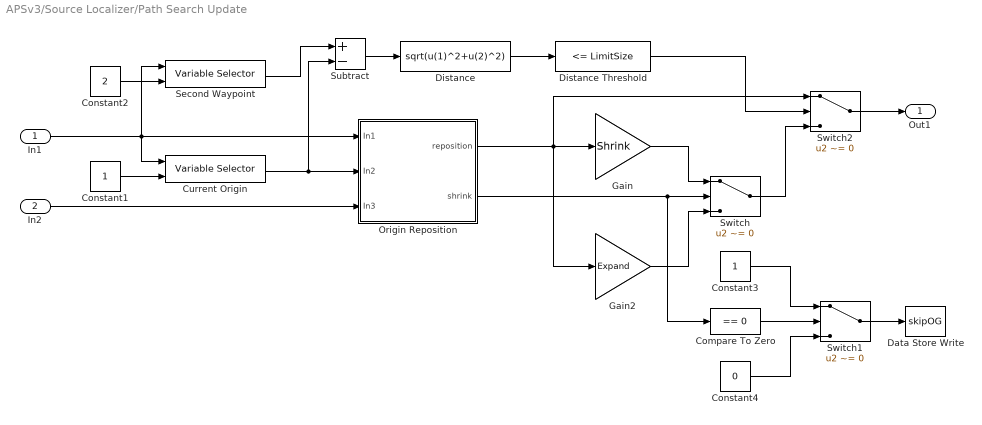
== system APSv3/Source Localizer/Path Search Update ==
  In1 : Inport
  In2 : Inport  Port=2
  Compare To Zero : simulink/Logic and Bit Operations/Compare To Zero  relop===  OutDataTypeStr=boolean
  Constant1 : Constant
  Constant2 : Constant  Value=2
  Constant3 : Constant
  Constant4 : Constant  Value=0
  Current Origin : dspindex/Variable Selector  NumInputs=1  rowsOrCols=Rows  IdxMode=Variable  Elements=[1 3]  ZerOneIdxMode=One-based  errmode=Clip Index  FillMode=off  FillValues=0
  Data Store Write : DataStoreWrite  DataStoreName=skipOG
  Distance : Fcn  Expr=sqrt(u(1)^2+u(2)^2)
  Distance Threshold : simulink/Logic and Bit Operations/Compare To Constant  relop=<=  const=LimitSize  OutDataTypeStr=boolean
  Gain : Gain  Gain=Shrink
  Gain2 : Gain  Gain=Expand
  Origin Reposition : Subsystem
  Second Waypoint : dspindex/Variable Selector  NumInputs=1  rowsOrCols=Rows  IdxMode=Variable  Elements=[1 3]  ZerOneIdxMode=One-based  errmode=Clip Index  FillMode=off  FillValues=0
  Subtract : Sum  Inputs=+-
  Switch : Switch  Criteria=u2 ~= 0  OutDataTypeStr=double  InputSameDT=on
  Switch1 : Switch  Criteria=u2 ~= 0  OutDataTypeStr=double  InputSameDT=on
  Switch2 : Switch  Criteria=u2 ~= 0  OutDataTypeStr=double  InputSameDT=on
  Out1 : Outport  VectorParamsAs1DForOutWhenUnconnected=off
  wires:
  In2/1 -> Origin Reposition/3(In3)
  Gain/1 -> Switch/1
  Gain2/1 -> Switch/3
  Switch/1 -> Switch2/3
  Origin Reposition/1(reposition) -> Switch2/1, Gain2/1, Gain/1
  In1/1 -> Second Waypoint/1, Current Origin/1, Origin Reposition/1(In1)
  Constant1/1 -> Current Origin/2
  Current Origin/1 -> Origin Reposition/2(In2), Subtract/2
  Origin Reposition/2(shrink) -> Compare To Zero/1, Switch/2
  Constant2/1 -> Second Waypoint/2
  Subtract/1 -> Distance/1
  Distance/1 -> Distance Threshold/1
  Second Waypoint/1 -> Subtract/1
  Distance Threshold/1 -> Switch2/2
  Switch2/1 -> Out1/1
  Compare To Zero/1 -> Switch1/2
  Switch1/1 -> Data Store Write/1
  Constant3/1 -> Switch1/1
  Constant4/1 -> Switch1/3

== system APSv3/Waypoint Goal Selector/Counter  ==
  In1 : Inport
  In2 : Inport  Port=2
  Counter : dspswit3/Counter  Direction=Up  CountEvent=Non-zero sample  CounterSize=User defined  MaxCount=255  InitialCount=1  Output=Count  HitValue=32  ResetInput=on  SamplesPerFrame=1  Ts=1  CntDtype=single  HitDtype=Logical
  Counter1 : dspswit3/Counter  Direction=Up  CountEvent=Rising edge  CounterSize=User defined  MaxCount=255  InitialCount=1  Output=Count  HitValue=32  ResetInput=on  SamplesPerFrame=1  Ts=1  CntDtype=double  HitDtype=Logical
  Detect Increase : simulink/Logic and Bit Operations/Detect Increase  vinit=0.0  OutDataTypeStr=boolean
  Out1 : Outport  VectorParamsAs1DForOutWhenUnconnected=off
  wires:
  In1/1 -> Counter/1
  Counter/1 -> Detect Increase/1
  Detect Increase/1 -> Counter1/1
  Counter1/1 -> Out1/1
  In2/1 -> Counter1/2, Counter/2

== system APSv3/Waypoint Goal Selector/Skip Conditions ==
  In1 : Inport
  Constant1 : Constant
  Counter : dspswit3/Counter  Direction=Up  CountEvent=Rising edge  CounterSize=User defined  MaxCount=255  InitialCount=0  Output=Count  HitValue=32  ResetInput=off  SamplesPerFrame=1  Ts=1  CntDtype=double  HitDtype=Logical
  Data Store Write4 : DataStoreWrite  DataStoreName=skip
  Ground1 : Ground
  Switch1 : Switch  Criteria=u2 > Threshold
  wires:
  Constant1/1 -> Switch1/1
  Counter/1 -> Switch1/2
  Switch1/1 -> Data Store Write4/1
  Ground1/1 -> Switch1/3
  In1/1 -> Counter/1

== system APSv3/Plume Simulator/Peak Selector/Reinitialize Cdet ==
  Constant : Constant  Value=MaxC
  Data Store Read3 : DataStoreRead  DataStoreName=Cdet
  Data Store Write2 : DataStoreWrite  DataStoreName=Cdet
  Ground2 : Ground
  Subtract : Sum  Inputs=-+
  Subtract1 : Sum  Inputs=-+
  Switch3 : Switch  Criteria=u2 > Threshold  OutDataTypeStr=double
  wires:
  Constant/1 -> Subtract/1
  Data Store Read3/1 -> Subtract/2, Subtract1/2
  Subtract/1 -> Switch3/1, Switch3/2
  Switch3/1 -> Subtract1/1
  Subtract1/1 -> Data Store Write2/1
  Ground2/1 -> Switch3/3

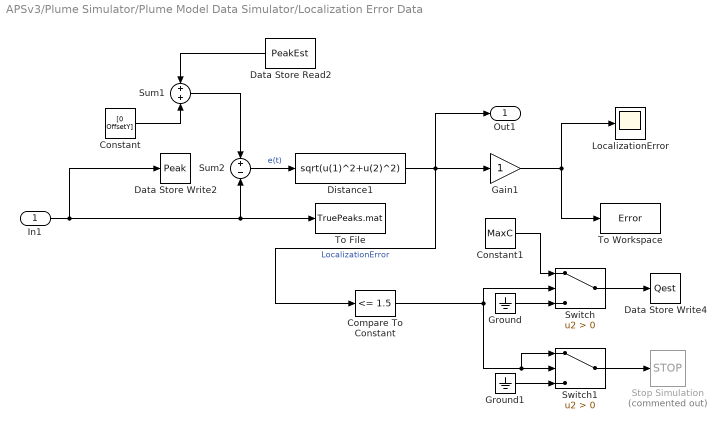
== system APSv3/Plume Simulator/Plume Model Data Simulator/Localization Error Data ==
  In1 : Inport
  Compare To Constant : simulink/Logic and Bit Operations/Compare To Constant  relop=<=  const=1.5  OutDataTypeStr=boolean
  Constant : Constant  Value=[0 OffsetY]
  Constant1 : Constant  Value=MaxC
  Data Store Read2 : DataStoreRead  DataStoreName=PeakEst
  Data Store Write2 : DataStoreWrite  DataStoreName=Peak
  Data Store Write4 : DataStoreWrite  DataStoreName=Qest
  Distance1 : Fcn  Expr=sqrt(u(1)^2+u(2)^2)
  Gain1 : Gain
  Ground : Ground
  Ground1 : Ground
  LocalizationError : Scope
  Stop Simulation : Stop  Commented=on
  Sum1 : Sum
  Sum2 : Sum  Inputs=+-
  Switch : Switch  Criteria=u2 > Threshold
  Switch1 : Switch  Criteria=u2 > Threshold
  To File : ToFile  Filename=TruePeaks.mat  MatrixName=ActualPeaks
      settings: Decimation=2
  To Workspace : ToWorkspace  VariableName=Error  SaveFormat=Timeseries  SampleTime=-1
  Out1 : Outport  VectorParamsAs1DForOutWhenUnconnected=off
  wires:
  Sum2/1 -> Distance1/1  "e(t)"
  Data Store Read2/1 -> Sum1/1
  Distance1/1 -> Out1/1, Compare To Constant/1, Gain1/1  "LocalizationError"
  In1/1 -> Data Store Write2/1, To File/1, Sum2/2
  Constant/1 -> Sum1/2
  Sum1/1 -> Sum2/1
  Gain1/1 -> To Workspace/1, LocalizationError/1
  Compare To Constant/1 -> Switch1/1, Switch1/2, Switch/2
  Ground/1 -> Switch/3
  Constant1/1 -> Switch/1
  Ground1/1 -> Switch1/3
  Switch1/1 -> Stop Simulation/1
  Switch/1 -> Data Store Write4/1

== system APSv3/Plume Simulator/Plume Model Data Simulator/Sensor Data Matrix ==
  In2 : Inport
  Constant : Constant  Value=N+1
  Constant1 : Constant  Value=PlumeD(:,:)
  Constant2 : Constant  Value=OffsetY
  Data Store Memory : DataStoreMemory  DataStoreName=maxPose  ReadBeforeWriteMsg=warning  WriteAfterWriteMsg=warning  WriteAfterReadMsg=warning  InitialValue=init  VectorParams1D=off  ShowAdditionalParam=off  OutDataTypeStr=double
  Data Store Read : DataStoreRead  DataStoreName=cMap
  Data Store Write : DataStoreWrite  DataStoreName=cMap
  MATLAB Function : MATLAB Function  TreatAsAtomicUnit=on
  Matrix Viewer : dspsnks4/Matrix Viewer  Commented=on  ImageParams=off  CMapStr=jet  AxisColorbar=on  AxisParams=off  AxisOrigin=Lower left corner  AxisTickMode=Auto  XTickRange=[0 150]  YTickRange=[0 50]  XLabel=X-axis  YLabel=Y-axis  ZLabel=Concentration  FigPos=get(0,'defaultfigureposition')  AxisZoom=off
      settings: SourceProductBaseCode=DS  YMin=0  YMax=MaxC
  Signal Specification : SignalSpecification  OutDataTypeStr=double  SampleTime=.01
  To Workspace : ToWorkspace  VariableName=cMap  SampleTime=-1
      settings: MaxDataPoints=100
  C : Outport  VectorParamsAs1DForOutWhenUnconnected=off
  MaxPose : Outport  Port=2  VectorParamsAs1DForOutWhenUnconnected=off
  wires:
  Constant/1 -> MATLAB Function/4(N)
  In2/1 -> MATLAB Function/3(poses)
  MATLAB Function/1(Cdata1) -> C/1
  Constant1/1 -> MATLAB Function/1(plume)
  Constant2/1 -> MATLAB Function/5(offY)
  Data Store Read/1 -> Signal Specification/1
  MATLAB Function/2(cMap1) -> To Workspace/1, Data Store Write/1, Matrix Viewer/1
  Signal Specification/1 -> MATLAB Function/2(cMap)
  MATLAB Function/3(MaxPose) -> MaxPose/1

== system APSv3/Plume Simulator/Plume Model Data Simulator/Sensor Positions ==
  In1 : Inport
  In2 : Inport  Port=2
  Radial Sensors : Subsystem
  Sensor Array : Subsystem
  Sensor Center : Subsystem
  Out1 : Outport  VectorParamsAs1DForOutWhenUnconnected=off
  Out2 : Outport  Port=2  VectorParamsAs1DForOutWhenUnconnected=off
  wires:
  In1/1 -> Radial Sensors/1(In1), Sensor Center/1(In2)
  In2/1 -> Radial Sensors/2(In2)
  Sensor Center/1(n) -> Sensor Array/1(In1)
  Sensor Center/2(Out1) -> Sensor Array/2(In2)
  Radial Sensors/1(Out1) -> Sensor Array/3(In3)
  Radial Sensors/2(Out2) -> Sensor Array/4(In4)
  Sensor Array/1(Out2) -> Out1/1
  Sensor Array/2(Out3) -> Out2/1

== system APSv3/Plume Simulator/Plume Model Data Simulator/Static Plume Concentrations ==
  Constant : Constant  Value=OffsetY
  Dynamic Plume Concentration Data : Constant  Value=PlumeD  VectorParams1D=off  OutDataTypeStr=double  LockScale=on
  MATLAB Function : MATLAB Function  TreatAsAtomicUnit=on
  Permute Dimensions1 : PermuteDimensions
  peak : Outport  VectorParamsAs1DForOutWhenUnconnected=off
  plume : Outport  Port=2  VectorParamsAs1DForOutWhenUnconnected=off
  wires:
  Dynamic Plume Concentration Data/1 -> MATLAB Function/1(PlumeD)
  MATLAB Function/1(Plume) -> Permute Dimensions1/1
  Permute Dimensions1/1 -> plume/1
  MATLAB Function/2(Peak) -> peak/1
  Constant/1 -> MATLAB Function/2(OffsetY)

== system APSv3/Plume Simulator/Plume Model Data Simulator/Subsystem ==
  In1 : Inport
  Constant : Constant
  Constant1 : Constant  Value=2
  Selector : Selector  InputPortWidth=2  IndexOptions=Index vector (port)  Indices=1  OutputSizes=1
  Selector2 : Selector  InputPortWidth=2  IndexOptions=Index vector (port)  Indices=1  OutputSizes=1
  Signal Specification1 : SignalSpecification  OutDataTypeStr=double  SampleTime=.01
  Vector Concatenate : Concatenate
  Out1 : Outport  VectorParamsAs1DForOutWhenUnconnected=off
  wires:
  Constant/1 -> Selector/2
  Vector Concatenate/1 -> Out1/1
  Constant1/1 -> Selector2/2
  Selector2/1 -> Vector Concatenate/2
  Signal Specification1/1 -> Selector/1, Selector2/1
  Selector/1 -> Vector Concatenate/1
  In1/1 -> Signal Specification1/1

== system APSv3/Skill Scores/Source Estimate (SQ)/Q estimate ==
  Constant : Constant  Value=MaxC
  Data Store Read : DataStoreRead  DataStoreName=Cdet
  Data Store Read1 : DataStoreRead  DataStoreName=Qest
  Data Store Read3 : DataStoreRead  DataStoreName=Qest
  Data Store Write2 : DataStoreWrite  DataStoreName=Qest
  Detect Increase : simulink/Logic and Bit Operations/Detect Increase  vinit=0.0  OutDataTypeStr=boolean
  Divide : Product  Inputs=*/
  Ground : Ground
  Relational Operator : RelationalOperator  OutDataTypeStr=boolean  RndMeth=Simplest
  Switch2 : Switch  Criteria=u2 > Threshold
  Switch3 : Switch  Criteria=u2 > Threshold
  To Workspace2 : ToWorkspace  VariableName=Qest  SaveFormat=Timeseries  SampleTime=-1
  wires:
  Ground/1 -> Switch2/3
  Detect Increase/1 -> Switch2/2
  Relational Operator/1 -> Switch3/2
  Switch2/1 -> Switch3/1, Relational Operator/1
  Data Store Read3/1 -> Switch3/3
  Switch3/1 -> Divide/1, Data Store Write2/1  "Estimated Maximum"
  Data Store Read1/1 -> Relational Operator/2
  Data Store Read/1 -> Switch2/1, Detect Increase/1  "<Gas Sensor>"
  Constant/1 -> Divide/2
  Divide/1 -> To Workspace2/1

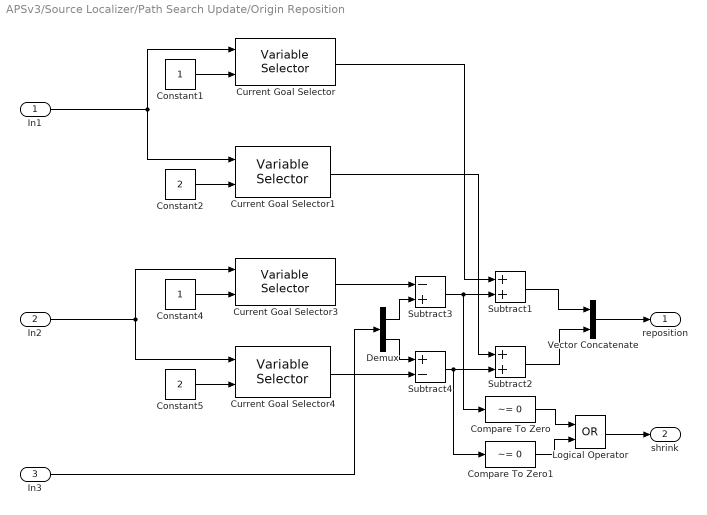
== system APSv3/Source Localizer/Path Search Update/Origin Reposition ==
  In1 : Inport
  In2 : Inport  Port=2
  In3 : Inport  Port=3
  Compare To Zero : simulink/Logic and Bit Operations/Compare To Zero  relop=~=  OutDataTypeStr=boolean
  Compare To Zero1 : simulink/Logic and Bit Operations/Compare To Zero  relop=~=  OutDataTypeStr=boolean
  Constant1 : Constant
  Constant2 : Constant  Value=2
  Constant4 : Constant
  Constant5 : Constant  Value=2
  Current Goal Selector{,1,3..4} (4 alike) : dspindex/Variable Selector  NumInputs=1  rowsOrCols=Columns  IdxMode=Variable  Elements=[1 3]  ZerOneIdxMode=One-based  errmode=Clip Index  FillMode=off  FillValues=0
  Demux : Demux  Outputs=2
  Logical Operator : Logic  Operator=OR  AllPortsSameDT=off  OutDataTypeStr=boolean
  Subtract1 : Sum
  Subtract2 : Sum
  Subtract3 : Sum  Inputs=-+
  Subtract4 : Sum  Inputs=+-
  Vector Concatenate : Concatenate  Mode=Multidimensional array  ConcatenateDimension=2
  reposition : Outport  VectorParamsAs1DForOutWhenUnconnected=off
  shrink : Outport  Port=2  VectorParamsAs1DForOutWhenUnconnected=off
  wires:
  In3/1 -> Demux/1
  Vector Concatenate/1 -> reposition/1
  Subtract1/1 -> Vector Concatenate/1
  In1/1 -> Current Goal Selector1/1, Current Goal Selector/1
  Current Goal Selector/1 -> Subtract1/1
  Constant1/1 -> Current Goal Selector/2
  Constant2/1 -> Current Goal Selector1/2
  Demux/1 -> Subtract3/2
  Current Goal Selector1/1 -> Subtract2/1
  Subtract2/1 -> Vector Concatenate/2
  Demux/2 -> Subtract4/1
  Constant4/1 -> Current Goal Selector3/2
  Constant5/1 -> Current Goal Selector4/2
  Current Goal Selector3/1 -> Subtract3/1
  Current Goal Selector4/1 -> Subtract4/2
  Subtract3/1 -> Compare To Zero/1, Subtract1/2
  Subtract4/1 -> Compare To Zero1/1, Subtract2/2
  In2/1 -> Current Goal Selector4/1, Current Goal Selector3/1
  Compare To Zero/1 -> Logical Operator/1
  Compare To Zero1/1 -> Logical Operator/2
  Logical Operator/1 -> shrink/1
